simulink model "TwoSwitchForward_Parta"  (R2018a)
settings: Solver=VariableStepAuto  StartTime=0.0  StopTime=0.01  RelTol=1e-3
libraries: powerlib x39
settings Model: Creator=Gulten  LastModifiedBy=Gulten

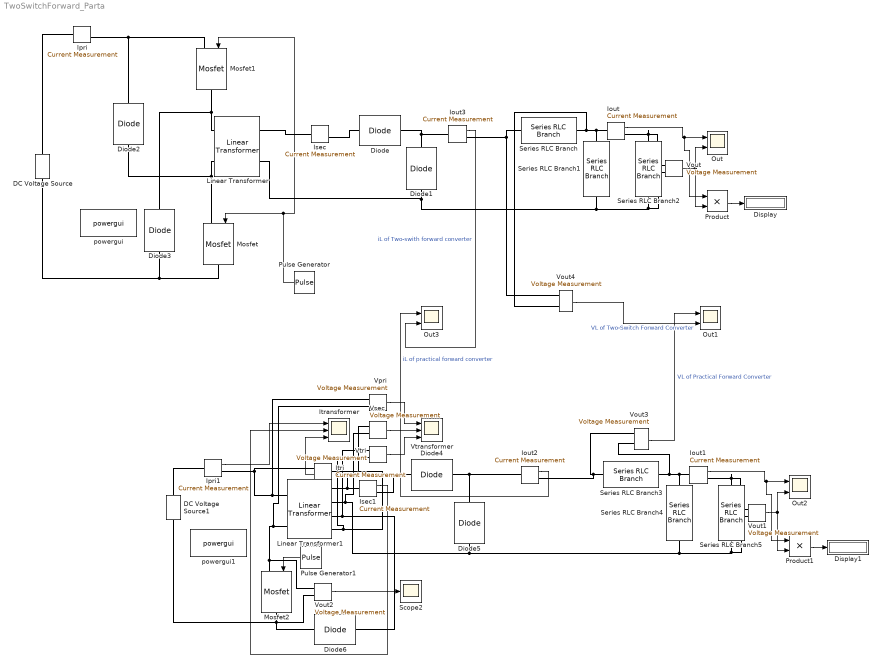
== system TwoSwitchForward_Parta ==
  DC Voltage Source : powerlib/Electrical Sources/DC Voltage Source  Amplitude=24  Measurements=None
  DC Voltage Source1 : powerlib/Electrical Sources/DC Voltage Source  Amplitude=24  Measurements=None
  Diode : powerlib/Power Electronics/Diode  Ron=0.001  Lon=0  Vf=0  IC=0  UseSnubber=0  Rs=500  Cs=250e-09  Measurements=off
  Diode{1..3,5..6} (5 alike) : powerlib/Power Electronics/Diode  Ron=0.001  Lon=0  Vf=0  IC=0  UseSnubber=0  Rs=500  Cs=250e-9  Measurements=off
  Diode4 : powerlib/Power Electronics/Diode  Ron=0.001  Lon=0  Vf=0  IC=0  UseSnubber=0  Rs=500  Cs=250e-09  Measurements=off
  Display : Display
  Display1 : Display
  Iout{,1..3} (4 alike) : powerlib/Measurements/Current Measurement  PhasorSimulation=off  OutputType=Complex  PSBequivalent=0
  Ipri : powerlib/Measurements/Current Measurement  PhasorSimulation=off  OutputType=Complex  PSBequivalent=0
  Ipri1 : powerlib/Measurements/Current Measurement  PhasorSimulation=off  OutputType=Complex  PSBequivalent=0
  Isec : powerlib/Measurements/Current Measurement  PhasorSimulation=off  OutputType=Complex  PSBequivalent=0
  Isec1 : powerlib/Measurements/Current Measurement  PhasorSimulation=off  OutputType=Complex  PSBequivalent=0
  Itransformer : Scope  NumInputPorts=3
  Itri : powerlib/Measurements/Current Measurement  PhasorSimulation=off  OutputType=Complex  PSBequivalent=0
  Linear Transformer : powerlib/Elements/Linear Transformer  UNITS=SI  NominalPower=[ 60 30000]  winding1=[24 0.015 1e-06]  winding2=[22 0.021044 1e-06]  ThreeWindings=off  winding3=[24 0.005 1e-06]  RmLm=[500 0.00076394]  Measurements=None  DataType=on
  Linear Transformer1 : powerlib/Elements/Linear Transformer  UNITS=SI  NominalPower=[ 60 30000]  winding1=[24 0.015 1e-06]  winding2=[22 0.021044 1e-06]  ThreeWindings=on  winding3=[24 0.005 1e-06]  RmLm=[500 0.00076394]  Measurements=None  DataType=on
  Mosfet : powerlib/Power Electronics/Mosfet  Ron=0.1  Lon=0  Rd=0.01  Vfd=0  IC=0  Rs=1e05  Cs=inf  Measurements=off
  Mosfet1 : powerlib/Power Electronics/Mosfet  Ron=0.1  Lon=0  Rd=0.01  Vfd=0  IC=0  Rs=1e05  Cs=inf  Measurements=off
  Mosfet2 : powerlib/Power Electronics/Mosfet  Ron=0.1  Lon=0  Rd=0.01  Vfd=0  IC=0  Rs=1e05  Cs=inf  Measurements=off
  Out{,1..3} (4 alike) : Scope  NumInputPorts=2
  Product : Product
  Product1 : Product
  Pulse Generator : DiscretePulseGenerator  PulseType=Time based  Period=0.000033  PulseWidth=50
  Pulse Generator1 : DiscretePulseGenerator  PulseType=Time based  Period=0.000033  PulseWidth=50
  Scope2 : Scope
  Series RLC Branch : powerlib/Elements/Series RLC Branch  LConnTagsString=__new0  RConnTagsString=__new0  BranchType=L  Resistance=1  Inductance=5e-4  SetiL0=off  InitialCurrent=0  Capacitance=1e-6  Setx0=off  InitialVoltage=0  Measurements=None
  Series RLC Branch1 : powerlib/Elements/Series RLC Branch  LConnTagsString=__new0  RConnTagsString=__new0  BranchType=C  Resistance=1  Inductance=1e-3  SetiL0=off  InitialCurrent=0  Capacitance=1e-5  Setx0=off  InitialVoltage=0  Measurements=None
  Series RLC Branch2 : powerlib/Elements/Series RLC Branch  LConnTagsString=__new0  RConnTagsString=__new0  BranchType=R  Resistance=2.5  Inductance=1e-3  SetiL0=off  InitialCurrent=0  Capacitance=1e-6  Setx0=off  InitialVoltage=0  Measurements=None
  Series RLC Branch3 : powerlib/Elements/Series RLC Branch  LConnTagsString=__new0  RConnTagsString=__new0  BranchType=L  Resistance=1  Inductance=5e-4  SetiL0=off  InitialCurrent=0  Capacitance=1e-6  Setx0=off  InitialVoltage=0  Measurements=None
  Series RLC Branch4 : powerlib/Elements/Series RLC Branch  LConnTagsString=__new0  RConnTagsString=__new0  BranchType=C  Resistance=1  Inductance=1e-3  SetiL0=off  InitialCurrent=0  Capacitance=1e-5  Setx0=off  InitialVoltage=0  Measurements=None
  Series RLC Branch5 : powerlib/Elements/Series RLC Branch  LConnTagsString=__new0  RConnTagsString=__new0  BranchType=R  Resistance=2.5  Inductance=1e-3  SetiL0=off  InitialCurrent=0  Capacitance=1e-6  Setx0=off  InitialVoltage=0  Measurements=None
  Vout{,1..4} (5 alike) : powerlib/Measurements/Voltage Measurement  PhasorSimulation=off  OutputType=Complex  PSBequivalent=0
  Vpri : powerlib/Measurements/Voltage Measurement  PhasorSimulation=off  OutputType=Complex  PSBequivalent=0
  Vsec : powerlib/Measurements/Voltage Measurement  PhasorSimulation=off  OutputType=Complex  PSBequivalent=0
  Vtransformer : Scope  NumInputPorts=3
  Vtri : powerlib/Measurements/Voltage Measurement  PhasorSimulation=off  OutputType=Complex  PSBequivalent=0
  powergui : powerlib/powergui  Priority=1  SimulationMode=Discrete  SampleTime=1e-8  frequency=60  Iterations=50  frequencyindice=0  Pbase=100e6  ErrMax=1e-4  UnitsV=kV  UnitsW=MW  buscounter=0  FunctionMessages=off  echomessages=off  EnableUseOfTLC=off  CurrentSourceSwitches=off  DisableSnubberDevices=off  DisableRonSwitches=off  DisableVfSwitches=off  DisplayEquations=off  SolverType=Tustin/Backward Euler (TBE)  Interpol=off  ExternalGateDelay=off  methode=off  Ts=100  x0status=blocks  SPID=on  SwTol=0  HookPort=off  RestoreLinks=warning  ResistiveCurrentMeasurement=off  Frange=[0:2:500]  Ylog=off  Xlog=on  ShowGrid=off  save=off  variable=ZData  structure=0  ZoomFFT=off  StartTime=0.0  cycles=1  DisplayStyle=1  fundamental=60  FreqAxis=off  MaxFrequency=1000  frequencyindicesteady=1  RmsSteady=1  display=off
  powergui1 : powerlib/powergui  Priority=1  SimulationMode=Discrete  SampleTime=1e-8  frequency=60  Iterations=50  frequencyindice=0  Pbase=100e6  ErrMax=1e-4  UnitsV=kV  UnitsW=MW  buscounter=0  FunctionMessages=off  echomessages=off  EnableUseOfTLC=off  CurrentSourceSwitches=off  DisableSnubberDevices=off  DisableRonSwitches=off  DisableVfSwitches=off  DisplayEquations=off  SolverType=Tustin/Backward Euler (TBE)  Interpol=off  ExternalGateDelay=off  methode=off  Ts=100  x0status=blocks  SPID=on  SwTol=0  HookPort=off  RestoreLinks=warning  ResistiveCurrentMeasurement=off  Frange=[0:2:500]  Ylog=off  Xlog=on  ShowGrid=off  save=off  variable=ZData  structure=0  ZoomFFT=off  StartTime=0.0  cycles=1  DisplayStyle=1  fundamental=60  FreqAxis=off  MaxFrequency=1000  frequencyindicesteady=1  RmsSteady=1  display=off
  wires:
  Vout/1 -> Product/2, Out/2
  Product/1 -> Display/1
  Iout/1 -> Product/1, Out/1
  Pulse Generator/1 -> Mosfet/1, Mosfet1/1
  Product1/1 -> Display1/1
  Iout1/1 -> Product1/1, Out2/1
  Vtri/1 -> Vtransformer/3
  Ipri1/1 -> Itransformer/1
  Vout1/1 -> Product1/2, Out2/2
  Pulse Generator1/1 -> Mosfet2/1
  Isec1/1 -> Itransformer/2
  Vsec/1 -> Vtransformer/2
  Itri/1 -> Itransformer/3
  Vpri/1 -> Vtransformer/1
  Vout2/1 -> Scope2/1
  Vout3/1 -> Out1/1  "VL of Practical Forward Converter"
  Vout4/1 -> Out1/2  "VL of Two-Switch Forward Converter"
  Iout3/1 -> Out3/2  "iL of Two-swith forward converter"
  Iout2/1 -> Out3/1  "iL of practical forward converter"
  connections:
  Diode1/LConn1 -- Linear Transformer/RConn2 -- Vout/LConn2 -- Series RLC Branch2/RConn1 -- Series RLC Branch1/RConn1
  Series RLC Branch2/LConn1 -- Iout/RConn1 -- Vout/LConn1
  Series RLC Branch/LConn1 -- Iout3/RConn1 -- Vout4/LConn1
  Series RLC Branch1/LConn1 -- Vout4/LConn2 -- Series RLC Branch/RConn1 -- Iout/LConn1
  Mosfet/RConn1 -- DC Voltage Source/LConn1 -- Diode3/LConn1
  Isec/LConn1 -- Linear Transformer/RConn1
  Isec/RConn1 -- Diode/LConn1
  DC Voltage Source/RConn1 -- Ipri/LConn1
  Ipri/RConn1 -- Diode2/RConn1 -- Mosfet1/LConn1
  Mosfet/LConn1 -- Diode2/LConn1 -- Linear Transformer/LConn2
  Mosfet1/RConn1 -- Diode3/RConn1 -- Linear Transformer/LConn1
  Linear Transformer1/RConn1 -- Isec1/LConn1 -- Vsec/LConn1
  Series RLC Branch3/RConn1 -- Vout3/LConn2 -- Iout1/LConn1 -- Series RLC Branch4/LConn1
  Diode5/RConn1 -- Iout2/LConn1 -- Diode4/RConn1
  Series RLC Branch5/LConn1 -- Iout1/RConn1 -- Vout1/LConn1
  Linear Transformer1/RConn3 -- Diode6/RConn1 -- Vtri/LConn1
  Itri/LConn1 -- Linear Transformer1/RConn4 -- Vtri/LConn2
  Diode5/LConn1 -- Linear Transformer1/RConn2 -- Vsec/LConn2 -- Series RLC Branch4/RConn1 -- Vout1/LConn2 -- Series RLC Branch5/RConn1
  Vout2/LConn2 -- Mosfet2/RConn1 -- Diode6/LConn1 -- DC Voltage Source1/LConn1
  Linear Transformer1/LConn1 -- Vpri/LConn1 -- Ipri1/RConn1 -- Itri/RConn1
  Vpri/LConn2 -- Linear Transformer1/LConn2 -- Vout2/LConn1 -- Mosfet2/LConn1
  Isec1/RConn1 -- Diode4/LConn1
  DC Voltage Source1/RConn1 -- Ipri1/LConn1
  Series RLC Branch3/LConn1 -- Iout2/RConn1 -- Vout3/LConn1
  Diode1/RConn1 -- Iout3/LConn1 -- Diode/RConn1
